simulink model "CBE_145_HW4_P4"  (R2020b)
settings: Solver=VariableStepAuto  StartTime=0.0  StopTime=10  RelTol=1e-3
settings Model: Creator=Jesus Vergara  LastModifiedBy=Jesus Vergara

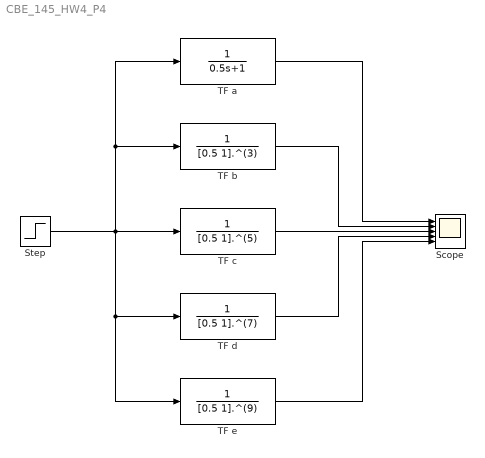
== system CBE_145_HW4_P4 ==
  Scope : Scope  NumInputPorts=5
  Step : Step  SampleTime=0
  "TF a " : TransferFcn  Denominator=[0.5 1]
  TF b : TransferFcn  Denominator=[0.5 1].^(3)
  TF c : TransferFcn  Denominator=[0.5 1].^(5)
  TF d : TransferFcn  Denominator=[0.5 1].^(7)
  TF e : TransferFcn  Denominator=[0.5 1].^(9)
  wires:
  "TF a "/1 -> Scope/1
  Step/1 -> TF b/1, "TF a "/1, TF e/1, TF d/1, TF c/1
  TF b/1 -> Scope/2
  TF c/1 -> Scope/3
  TF d/1 -> Scope/4
  TF e/1 -> Scope/5
